simulink model "move_forward_hardware"  (R2021a)
settings: Solver=FixedStepDiscrete  StartTime=0.0  StopTime=5  FixedStep=0.01  RelTol=1e-3
undefined symbols (not defined in the file): InputPWM, ticksPerRot, wheelR, WheelSpeed
libraries: arduinolib x6, spsEdgeDetectorLib x2, pid_lib x1, mobileRoboticsTrainingLib x1
settings Model: SILPILModeSetting=veronly  EnablePacing=on  ExtModeTrigDuration=2  Creator=Boitumelo  LastModifiedBy=markl
settings OptimizationCC: EnhancedBackFolding=on  PassReuseOutputArgsAs=Individual arguments  ZeroExternalMemoryAtStartup=off  ZeroInternalMemoryAtStartup=off  MaxStackSize=64  OptimizeBlockOrder=speed  DifferentSizesBufferReuse=on  OptimizationCustomize=off  EfficientTunableParamExpr=on
settings DebuggingCC: ParameterTunabilityLossMsg=error
settings HardwareCC: ProdBitPerInt=16  ProdBitPerPointer=16  ProdBitPerSizeT=16  ProdBitPerPtrDiffT=16  ProdLargestAtomicFloat=None  ProdWordSize=8  ProdHWDeviceType=Atmel->AVR  UseEmbeddedCoderFeatures=off  UseSimulinkCoderFeatures=off
settings SFSimCC: MATLABDynamicMemAlloc=off
settings RTWCC: SystemTargetFile=ert.tlc  HardwareBoard=Arduino Leonardo  TemplateMakefile=ert_default_tmf  Toolchain=Arduino AVR
settings CodeAppCC: ForceParamTrailComments=on  IgnoreCustomStorageClasses=off  OperatorAnnotations=on  SimulinkDataObjDesc=on  SFDataObjDesc=on  InsertBlockDesc=on
settings ERTTargetCC: SupportContinuousTime=on  SupportNonInlinedSFcns=on  SupportVariableSizeSignals=on  ExtModeTransport=5  ExtModeStaticAllocSize=250  ExtModeMexFile=ext_serial_win32_comm_leonardo

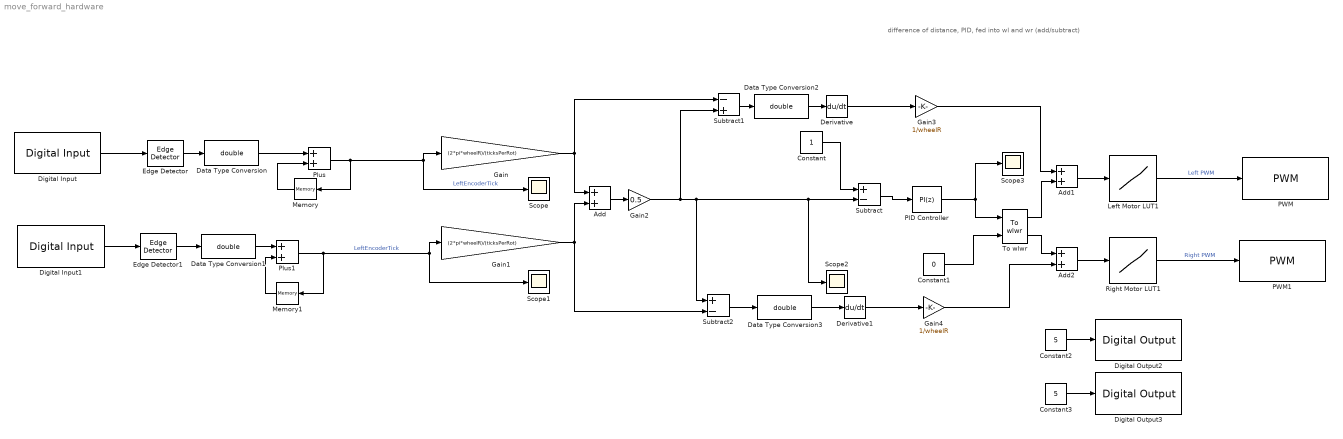
== system move_forward_hardware ==
  note: difference of distance, PID, fed into wl and wr (add/subtract)
  Add : Sum
  Add1 : Sum
  Add2 : Sum
  Constant : Constant
  Constant1 : Constant  Value=0
  Constant2 : Constant  Value=5
  Constant3 : Constant  Value=5
  Data Type Conversion{,1..3} (4 alike) : DataTypeConversion  OutDataTypeStr=double
  Derivative : Derivative
  Derivative1 : Derivative
  Digital Input : arduinolib/Digital Input  pinNumber=2  mode=Default  Direction=input  SampleTime=0.01  blockPlatform=arduino
  Digital Input1 : arduinolib/Digital Input  pinNumber=3  mode=Default  Direction=input  SampleTime=0.01  blockPlatform=arduino
  Digital Output2 : arduinolib/Digital Output  pinNumber=4  Direction=output  blockPlatform=arduino
  Digital Output3 : arduinolib/Digital Output  pinNumber=7  Direction=output  blockPlatform=arduino
  Edge Detector : spsEdgeDetectorLib/Edge Detector  model=Either  ic=0  Ts=0
      settings: SourceProductBaseCode=PS
  Edge Detector1 : spsEdgeDetectorLib/Edge Detector  model=Either  ic=0  Ts=0
      settings: SourceProductBaseCode=PS
  Gain : Gain  Gain=(2*pi*wheelR)/(ticksPerRot)
  Gain1 : Gain  Gain=(2*pi*wheelR)/(ticksPerRot)
  Gain2 : Gain  Gain=0.5
  Gain3 : Gain  Gain=1/wheelR
  Gain4 : Gain  Gain=1/wheelR
  Left Motor LUT1 : Lookup_n-D  NumberOfTableDimensions=1  BreakpointsForDimension1=WheelSpeed  Table=InputPWM  InterpMethod=Nearest  ExtrapMethod=Clip  InternalRulePriority=Speed  RndMeth=Simplest  InputSameDT=on
  Memory : Memory
  Memory1 : Memory
  PID Controller : pid_lib/PID Controller  Controller=PI  Form=Parallel  TimeDomain=Discrete-time  UseExternalTs=off  SampleTime=-1  IntegratorMethod=Forward Euler  FilterMethod=Forward Euler  ControllerParametersSource=internal  P=5  I=0.1  D=0.1  UseFilter=on  N=100  TunerSelectOption=Transfer Function Based (PID Tuner App)  InitialConditionSource=internal  InitialConditionForIntegrator=0  InitialConditionForFilter=0  DifferentiatorICPrevScaledInput=0  ExternalReset=none  TrackingMode=off  Kt=1  LimitOutput=on  SatLimitsSource=internal  UpperSaturationLimit=12.5601  LowerSaturationLimit=-12.5601  LinearizeAsGain=on  AntiWindupMode=clamping  Kb=1  POutMin=[]  POutMax=[]  IOutMin=[]  IOutMax=[]  DOutMin=[]  DOutMax=[]  NOutMin=[]  NOutMax=[]  SumOutMin=[]  SumOutMax=[]  SaturationOutMin=[]  SaturationOutMax=[]  PParamMin=[]  PParamMax=[]  IParamMin=[]  IParamMax=[]  DParamMin=[]  DParamMax=[]  NParamMin=[]  NParamMax=[]  KbParamMin=[]  KbParamMax=[]  KtParamMin=[]  KtParamMax=[]  KbOutMin=[]  KbOutMax=[]  KtOutMin=[]  KtOutMax=[]  IntegratorOutMin=[]  IntegratorOutMax=[]  FilterOutMin=[]  FilterOutMax=[]  SumI1OutMin=[]  SumI1OutMax=[]  SumI2OutMin=[]  SumI2OutMax=[]  SumI3OutMin=[]  SumI3OutMax=[]  SumI4OutMin=[]  SumI4OutMax=[]  SumDOutMin=[]  SumDOutMax=[]  DifferentiatorOutMin=[]  DifferentiatorOutMax=[]  FilterDiffOutCoefMin=[]  FilterDiffOutCoefMax=[]  ReciprocalOutMin=[]  ReciprocalOutMax=[]  SumDenOutMin=[]  SumDenOutMax=[]  SumNumOutMin=[]  SumNumOutMax=[]  DivideOutMin=[]  DivideOutMax=[]  UdiffTsProdOutMin=[]  UdiffTsProdOutMax=[]  NTsProdOutMin=[]  NTsProdOutMax=[]  UintegralTsProdOutMin=[]  UintegralTsProdOutMax=[]  UngainTsProdOutMin=[]  UngainTsProdOutMax=[]  IntegratorContinuousStateAttributes=''  IntegratorStateMustResolveToSignalObject=off  IntegratorRTWStateStorageClass=Auto  FilterContinuousStateAttributes=''  FilterStateMustResolveToSignalObject=off  FilterRTWStateStorageClass=Auto  ParallelPVariant=InternalParameters  IdealPVariant=Disabled  IVariant=InternalParameters  DVariant=Disabled  IntegratorVariant=Discrete  SatVariant=Enabled  AWVariant=DiscClampingParallel  PCopyVariant=Disabled  TRVariant=Disabled  FdbkBlocksVariant=Forward  IdealPFdbkVariant=Disabled  SatFdbkVariant=Disabled  DerivativeFilterVariant=Disabled  NVariant=Disabled  NCopyVariant=Disabled_SignalSpec  FilterICVariant=Disabled  IntegratorICVariant=InternalICs  ExternalResetVariant=Disabled  TRSumVariant=Passthrough  SumFdbkVariant=Disabled  SumVariant=Sum_PI  TsampFilterVariant=InternalTs  TsampNgainVariant=Passthrough  TsampIntegralVariant=Passthrough  ExternalSaturationOutDataTypeStr=Inherit: Same as second input  InitialConditionSetting=Output
  PWM : arduinolib/PWM  pinNumber=5  frequencyType=Default  desiredFrequency=490.2  achievableFrequency=490.2
  PWM1 : arduinolib/PWM  pinNumber=6  frequencyType=Default  desiredFrequency=490.2  achievableFrequency=490.2
  Plus : Sum
  Plus1 : Sum
  Right Motor LUT1 : Lookup_n-D  NumberOfTableDimensions=1  BreakpointsForDimension1=WheelSpeed  Table=InputPWM  InterpMethod=Nearest  ExtrapMethod=Clip  InternalRulePriority=Speed  RndMeth=Simplest  InputSameDT=on
  Scope{,1..3} (4 alike) : Scope
  Subtract : Sum  Inputs=+-
  Subtract1 : Sum  Inputs=-+
  Subtract2 : Sum  Inputs=+-
  To wlwr : mobileRoboticsTrainingLib/To wlwr  axleLength=axleLength  wheelR=wheelR
  wires:
  Plus/1 -> Memory/1, Gain/1, Scope/1  "LeftEncoderTick"
  Gain/1 -> Add/1, Subtract1/1
  Gain1/1 -> Add/2, Subtract2/2
  Add/1 -> Gain2/1
  Gain2/1 -> Subtract1/2, Subtract2/1, Scope2/1, Subtract/2
  PID Controller/1 -> Scope3/1, To wlwr/1
  Constant1/1 -> To wlwr/2
  Constant/1 -> Subtract/1
  Subtract/1 -> PID Controller/1
  Digital Input/1 -> Edge Detector/1
  Edge Detector/1 -> Data Type Conversion/1
  Digital Input1/1 -> Edge Detector1/1
  Constant2/1 -> Digital Output2/1
  Constant3/1 -> Digital Output3/1
  Add1/1 -> Left Motor LUT1/1
  Add2/1 -> Right Motor LUT1/1
  Left Motor LUT1/1 -> PWM/1  "Left PWM"
  Right Motor LUT1/1 -> PWM1/1  "Right PWM"
  Memory/1 -> Plus/2
  Data Type Conversion/1 -> Plus/1
  Memory1/1 -> Plus1/2
  Plus1/1 -> Memory1/1, Gain1/1, Scope1/1  "LeftEncoderTick"
  Data Type Conversion1/1 -> Plus1/1
  Edge Detector1/1 -> Data Type Conversion1/1
  To wlwr/1 -> Add1/2
  Derivative/1 -> Gain3/1
  Derivative1/1 -> Gain4/1
  To wlwr/2 -> Add2/1
  Gain3/1 -> Add1/1
  Gain4/1 -> Add2/2
  Subtract1/1 -> Data Type Conversion2/1
  Data Type Conversion2/1 -> Derivative/1
  Data Type Conversion3/1 -> Derivative1/1
  Subtract2/1 -> Data Type Conversion3/1
